simulink model "SF107A_MotRplCoggCmd"  (R2013b)
settings: Solver=FixedStepDiscrete  SolverMode=SingleTasking  StartTime=0.0  StopTime=1  FixedStep=0.002  RelTol=1e-3
values from neighbouring files (symbols this model uses):
  ARCHGLBPRM_2PI_ULS_F32 = DataDict.Constant    [SF107A_MotRplCoggCmd_DataDict.m]
  ARCHGLBPRM_FLOATZEROTHD_ULS_F32 = DataDict.Constant    [SF107A_MotRplCoggCmd_DataDict.m]
  ININITRNIDXCON_CNT_U16 = DataDict.Constant    [SF107A_MotRplCoggCmd_DataDict.m]
  ITRNIDXCON_CNT_U08 = DataDict.Constant    [SF107A_MotRplCoggCmd_DataDict.m]
  MotRplCoggCmdHrmncOrder1Elec = DataDict.Calibration    [SF107A_MotRplCoggCmd_DataDict.m]
  MotRplCoggCmdHrmncOrder2Elec = DataDict.Calibration    [SF107A_MotRplCoggCmd_DataDict.m]
  MotRplCoggCmdHrmncOrder3Elec = DataDict.Calibration    [SF107A_MotRplCoggCmd_DataDict.m]
  ONEOVER12_MOTREV_F32 = DataDict.Constant    [SF107A_MotRplCoggCmd_DataDict.m]
  ONEOVER2_ULS_F32 = DataDict.Constant    [SF107A_MotRplCoggCmd_DataDict.m]
  ONEOVER2PI_ULS_F32 = DataDict.Constant    [SF107A_MotRplCoggCmd_DataDict.m]
  ONEOVER4_ULS_F32 = DataDict.Constant    [SF107A_MotRplCoggCmd_DataDict.m]
  SINCNVNCON1_ULS_F32 = DataDict.Constant    [SF107A_MotRplCoggCmd_DataDict.m]
  SINCNVNCON2_ULS_F32 = DataDict.Constant    [SF107A_MotRplCoggCmd_DataDict.m]
  SINCNVNCONTBL_ULS_U16 = DataDict.Constant    [SF107A_MotRplCoggCmd_DataDict.m]
undefined symbols (not defined in the file or in its folder): NvmGetErrSts1
libraries: FloatToFixd x8, FixdToFloat x8, NxtrNvM x3, NxtrLim x3, simulink x2, NxtrAbslt x1
(part 2 of 3)

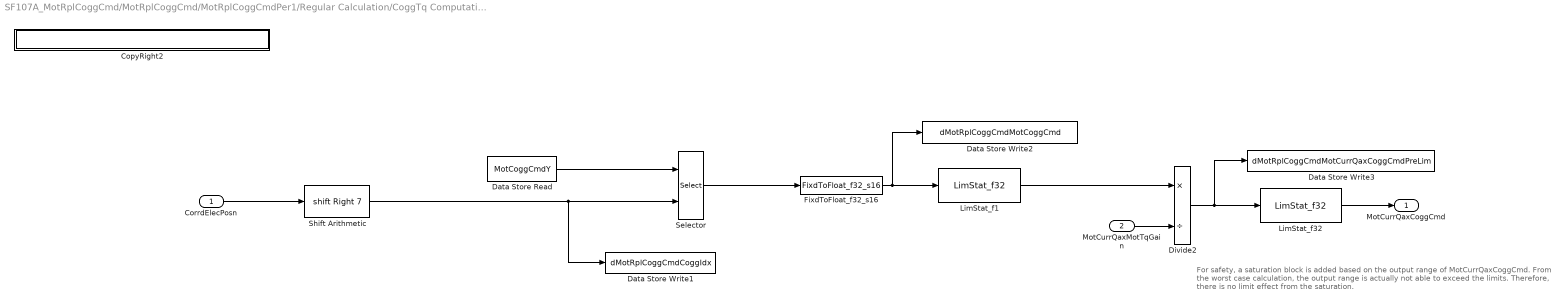
== system SF107A_MotRplCoggCmd/MotRplCoggCmd/MotRplCoggCmdPer1/Regular Calculation/CoggTq Computation ==
  note: For safety, a saturation block is added based on the output range of MotCurrQaxCoggCmd.
      | From the worst case calculation, the output range is actually not able to exceed the limits.
      | Therefore, there is no limit effect from the saturation.
  CorrdElecPosn : Inport
  MotCurrQaxMotTqGain : Inport  Port=2
  CopyRight2 : Subsystem  Description=|  mask(Copyright Information){none=on}
      | Copyright info block.                                               
      |                                                                     
      | Place copyright information at the top of every subsystem in design.
      mask prompts: none "No parameters"
      mask help: Place copyright information at the top of every subsystem in design.
      mask Display:
      | NxtrConf = 'Nexteer Confidential';
      | 
      | sys = bdroot; %handle for the current model ("system")
      | first = get_param(sys,'Created');
      | if(isempty(first))
      |     first = datestr(now,'yyyy');
      | else
      |     first = first(end-3:end);  %year is last four digits
      | end
      | 
      | last = get_param(sys,'LastModifiedDate');
      | if isempty(last)
      |     last = datestr(now,'yyyy');
      | else
      |     last = last(end-3:end);
      | end
      | 
      | if strcmp(first,last)
      |     fprintf('%s -- Copyright %s Nexteer',NxtrConf,first)
      | else
      |     fprintf('%s -- %s%s- %s Nexteer',NxtrConf,char(169),first,last)
      | end
  Data Store Read : DataStoreRead  RequirementInfo="{'linktype_rmi_doors' '0000bb46 (/E-STEER Core/SubSystem Specifications/Application Functions/SF99/SF107A Cogging and Ripple Command Generation)' '#SF107A_56' 'true' 'REQ:  SF107A_56' '' } %GIDa_3e95ac0e_f3f3_418f_9ebe_c4c5a1a291e1"  DataStoreName=MotCoggCmdY
  Data Store Write1 : DataStoreWrite  DataStoreName=dMotRplCoggCmdCoggIdx
  Data Store Write2 : DataStoreWrite  DataStoreName=dMotRplCoggCmdMotCoggCmd
  Data Store Write3 : DataStoreWrite  DataStoreName=dMotRplCoggCmdMotCurrQaxCoggCmdPreLim
  Divide2 : Product  RequirementInfo="{'linktype_rmi_doors' '0000bb46 (/E-STEER Core/SubSystem Specifications/Application Functions/SF99/SF107A Cogging and Ripple Command Generation)' '#SF107A_59' 'true' 'REQ:  SF107A_59' '' } %GIDa_3d8574ba_c11a_41bc_960f_b43c967fb16a"  Inputs=*/
  FixdToFloat_f32_s16 : FixdToFloat/FixdToFloat_f32_s16  Param1=14
  LimStat_f1 : NxtrLim/LimStat_f32  RequirementInfo="{'linktype_rmi_doors' '0000bb46 (/E-STEER Core/SubSystem Specifications/Application Functions/SF99/SF107A Cogging and Ripple Command Generation)' '#SF107A_52' 'true' 'REQ:  SF107A_52' '' } %GIDa_e794c357_2251_4144_9bb5_41f34ca7d615"  LoLim=MOTCOGGCMDLOLIM_MOTNWTMTR_F32  HiLim=MOTCOGGCMDHILIM_MOTNWTMTR_F32
      settings: AttributesFormatString=|
      | Low Limit: %<LoLim>
      | High Limit:%<HiLim>
  LimStat_f32 : NxtrLim/LimStat_f32  LoLim=MOTCURRCOGGCMDLOLIM_AMPR_F32  HiLim=MOTCURRCOGGCMDHILIM_AMPR_F32
      settings: AttributesFormatString=|
      | Low Limit: %<LoLim>
      | High Limit:%<HiLim>
  Selector : Selector  IndexMode=Zero-based  InputPortWidth=512  IndexOptions=Index vector (port)  Indices=[1 3]  OutputSizes=1
  Shift Arithmetic : ArithShift  BitShiftNumber=7  BitShiftDirection=Right
  MotCurrQaxCoggCmd : Outport
  wires:
  Selector/1 -> FixdToFloat_f32_s16/1
  FixdToFloat_f32_s16/1 -> LimStat_f1/1, Data Store Write2/1
  Data Store Read/1 -> Selector/1
  CorrdElecPosn/1 -> Shift Arithmetic/1
  MotCurrQaxMotTqGain/1 -> Divide2/2
  Divide2/1 -> LimStat_f32/1, Data Store Write3/1
  LimStat_f32/1 -> MotCurrQaxCoggCmd/1
  LimStat_f1/1 -> Divide2/1
  Shift Arithmetic/1 -> Data Store Write1/1, Selector/2

== system SF107A_MotRplCoggCmd/MotRplCoggCmd/MotRplCoggCmdPer1/Regular Calculation/CopyRight2 ==

== system SF107A_MotRplCoggCmd/MotRplCoggCmd/MotRplCoggCmdPer1/Regular Calculation/MotElecMeclPolarity Compensating ==
  MotElecMeclPolarity : Inport
  CopyRight2 : Subsystem  Description=|  mask(Copyright Information){none=on}
      | Copyright info block.                                               
      |                                                                     
      | Place copyright information at the top of every subsystem in design.
      mask prompts: none "No parameters"
      mask help: Place copyright information at the top of every subsystem in design.
      mask Display:
      | NxtrConf = 'Nexteer Confidential';
      | 
      | sys = bdroot; %handle for the current model ("system")
      | first = get_param(sys,'Created');
      | if(isempty(first))
      |     first = datestr(now,'yyyy');
      | else
      |     first = first(end-3:end);  %year is last four digits
      | end
      | 
      | last = get_param(sys,'LastModifiedDate');
      | if isempty(last)
      |     last = datestr(now,'yyyy');
      | else
      |     last = last(end-3:end);
      | end
      | 
      | if strcmp(first,last)
      |     fprintf('%s -- Copyright %s Nexteer',NxtrConf,first)
      | else
      |     fprintf('%s -- %s%s- %s Nexteer',NxtrConf,char(169),first,last)
      | end
  If1 : If  RequirementInfo="{'linktype_rmi_doors' '0000bb46 (/E-STEER Core/SubSystem Specifications/Application Functions/SF99/SF107A Cogging and Ripple Command Generation)' '#SF107A_48' 'true' 'REQ:  SF107A_48' '' } %GIDa_a3654d20_efbd_409e_83f9_fffa28f30d15"  IfExpression=u1==1
  Merge1 : Merge  RequirementInfo="{'linktype_rmi_doors' '0000bb46 (/E-STEER Core/SubSystem Specifications/Application Functions/SF99/SF107A Cogging and Ripple Command Generation)' '#SF107A_48' 'true' 'REQ:  SF107A_48' '' } %GIDa_23ad6171_7acd_41c2_a6a2_32a771c6a2a5"
  Output -1/12 MotRev : Subsystem  RequirementInfo="{'linktype_rmi_doors' '0000bb46 (/E-STEER Core/SubSystem Specifications/Application Functions/SF99/SF107A Cogging and Ripple Command Generation)' '#SF107A_48' 'true' 'REQ:  SF107A_48' '' } %GIDa_8d1ad6c2_c515_4934_932f_4d33d8ad8416"  TreatAsAtomicUnit=on
  Output 1/12 MotRev : Subsystem  RequirementInfo="{'linktype_rmi_doors' '0000bb46 (/E-STEER Core/SubSystem Specifications/Application Functions/SF99/SF107A Cogging and Ripple Command Generation)' '#SF107A_48' 'true' 'REQ:  SF107A_48' '' } %GIDa_3ad96f2a_4308_4c62_b762_7be6e9bb4790"  TreatAsAtomicUnit=on
  MotElecMeclPolarityCmp : Outport
  wires:
  If1/2 -> Output 1/12 MotRev/Action
  MotElecMeclPolarity/1 -> If1/1
  Merge1/1 -> MotElecMeclPolarityCmp/1
  Output -1/12 MotRev/1(Out1) -> Merge1/1
  If1/1 -> Output -1/12 MotRev/Action
  Output 1/12 MotRev/1(Out1) -> Merge1/2

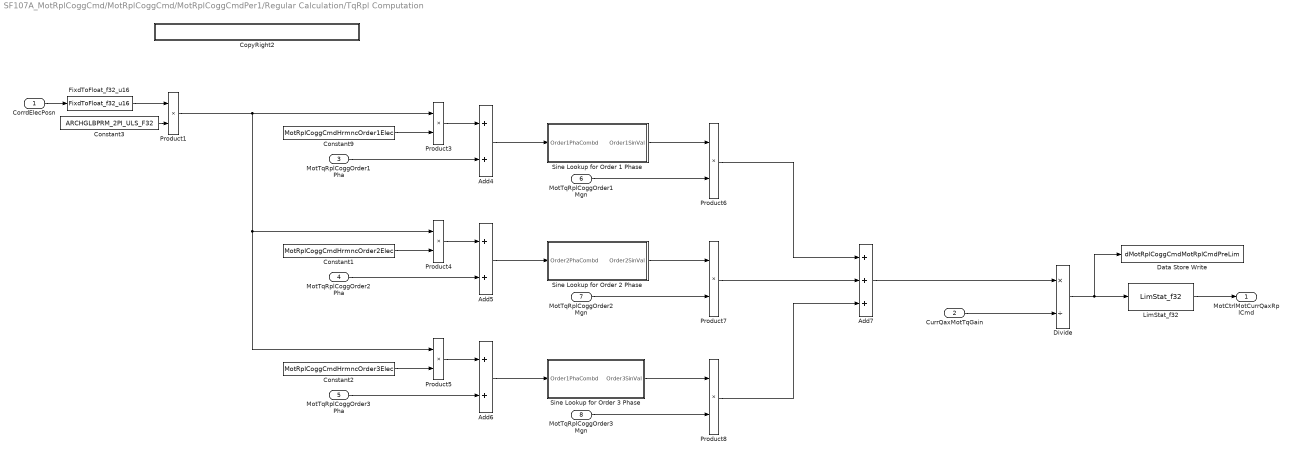
== system SF107A_MotRplCoggCmd/MotRplCoggCmd/MotRplCoggCmdPer1/Regular Calculation/TqRpl Computation ==
  CorrdElecPosn : Inport
  CurrQaxMotTqGain : Inport  Port=2
  MotTqRplCoggOrder1Pha : Inport  Port=3
  MotTqRplCoggOrder2Pha : Inport  Port=4
  MotTqRplCoggOrder3Pha : Inport  Port=5
  MotTqRplCoggOrder1Mgn : Inport  Port=6
  MotTqRplCoggOrder2Mgn : Inport  Port=7
  MotTqRplCoggOrder3Mgn : Inport  Port=8
  Add4 : Sum  RequirementInfo="{'linktype_rmi_doors' '0000bb46 (/E-STEER Core/SubSystem Specifications/Application Functions/SF99/SF107A Cogging and Ripple Command Generation)' '#SF107A_55' 'true' 'REQ:  SF107A_55' '' } %GIDa_c2399abb_93fd_4ea1_98cc_b0680e968892"
  Add5 : Sum  RequirementInfo="{'linktype_rmi_doors' '0000bb46 (/E-STEER Core/SubSystem Specifications/Application Functions/SF99/SF107A Cogging and Ripple Command Generation)' '#SF107A_55' 'true' 'REQ:  SF107A_55' '' } %GIDa_b4420672_1f55_4f94_87a8_96d9d357a965"
  Add6 : Sum  RequirementInfo="{'linktype_rmi_doors' '0000bb46 (/E-STEER Core/SubSystem Specifications/Application Functions/SF99/SF107A Cogging and Ripple Command Generation)' '#SF107A_55' 'true' 'REQ:  SF107A_55' '' } %GIDa_2dfbb206_2493_4fc1_9000_00a8fdd76cd7"
  Add7 : Sum  RequirementInfo="{'linktype_rmi_doors' '0000bb46 (/E-STEER Core/SubSystem Specifications/Application Functions/SF99/SF107A Cogging and Ripple Command Generation)' '#SF107A_54' 'true' 'REQ:  SF107A_54' '' } %GIDa_a8f048de_6f77_4343_a15f_fc7051edaaac"  Inputs=+++
  Constant1 : Constant  RequirementInfo="{'linktype_rmi_doors' '0000bb46 (/E-STEER Core/SubSystem Specifications/Application Functions/SF99/SF107A Cogging and Ripple Command Generation)' '#SF107A_57' 'true' 'REQ:  SF107A_57' '' } %GIDa_b7ef4c69_0a2c_4e9d_b8a7_dfaab4ba9f27"  Value=MotRplCoggCmdHrmncOrder2Elec
  Constant2 : Constant  RequirementInfo="{'linktype_rmi_doors' '0000bb46 (/E-STEER Core/SubSystem Specifications/Application Functions/SF99/SF107A Cogging and Ripple Command Generation)' '#SF107A_57' 'true' 'REQ:  SF107A_57' '' } %GIDa_07332141_8940_47cd_a6c0_7085309b4753"  Value=MotRplCoggCmdHrmncOrder3Elec
  Constant3 : Constant  Value=ARCHGLBPRM_2PI_ULS_F32
  Constant9 : Constant  RequirementInfo="{'linktype_rmi_doors' '0000bb46 (/E-STEER Core/SubSystem Specifications/Application Functions/SF99/SF107A Cogging and Ripple Command Generation)' '#SF107A_57' 'true' 'REQ:  SF107A_57' '' } %GIDa_3c0a14e8_7767_4d2c_90ce_8f5a73270d9c"  Value=MotRplCoggCmdHrmncOrder1Elec
  CopyRight2 : Subsystem  Description=|  mask(Copyright Information){none=on}
      | Copyright info block.                                               
      |                                                                     
      | Place copyright information at the top of every subsystem in design.
      mask prompts: none "No parameters"
      mask help: Place copyright information at the top of every subsystem in design.
      mask Display:
      | NxtrConf = 'Nexteer Confidential';
      | 
      | sys = bdroot; %handle for the current model ("system")
      | first = get_param(sys,'Created');
      | if(isempty(first))
      |     first = datestr(now,'yyyy');
      | else
      |     first = first(end-3:end);  %year is last four digits
      | end
      | 
      | last = get_param(sys,'LastModifiedDate');
      | if isempty(last)
      |     last = datestr(now,'yyyy');
      | else
      |     last = last(end-3:end);
      | end
      | 
      | if strcmp(first,last)
      |     fprintf('%s -- Copyright %s Nexteer',NxtrConf,first)
      | else
      |     fprintf('%s -- %s%s- %s Nexteer',NxtrConf,char(169),first,last)
      | end
  Data Store Write : DataStoreWrite  DataStoreName=dMotRplCoggCmdMotRplCmdPreLim
  Divide : Product  RequirementInfo="{'linktype_rmi_doors' '0000bb46 (/E-STEER Core/SubSystem Specifications/Application Functions/SF99/SF107A Cogging and Ripple Command Generation)' '#SF107A_53' 'true' 'REQ:  SF107A_53' '' } %GIDa_9f56ecef_e0c7_4e4a_ab4c_0d70a2d29558"  Inputs=*/
  FixdToFloat_f32_u16 : FixdToFloat/FixdToFloat_f32_u16  Param1=16
  LimStat_f32 : NxtrLim/LimStat_f32  LoLim=MOTRPLCMDLOLIM_AMPR_F32  HiLim=MOTRPLCMDHILIM_AMPR_F32
      settings: AttributesFormatString=|
      | Low Limit: %<LoLim>
      | High Limit:%<HiLim>
  Product1 : Product  RequirementInfo="{'linktype_rmi_doors' '0000bb46 (/E-STEER Core/SubSystem Specifications/Application Functions/SF99/SF107A Cogging and Ripple Command Generation)' '#SF107A_55' 'true' 'REQ:  SF107A_55' '' } %GIDa_8be27b70_a591_415b_b0b6_be9767e7231d"
  Product3 : Product  RequirementInfo="{'linktype_rmi_doors' '0000bb46 (/E-STEER Core/SubSystem Specifications/Application Functions/SF99/SF107A Cogging and Ripple Command Generation)' '#SF107A_55' 'true' 'REQ:  SF107A_55' '' } %GIDa_dd8066b3_0179_4f2f_b312_accdda934f40"
  Product4 : Product  RequirementInfo="{'linktype_rmi_doors' '0000bb46 (/E-STEER Core/SubSystem Specifications/Application Functions/SF99/SF107A Cogging and Ripple Command Generation)' '#SF107A_55' 'true' 'REQ:  SF107A_55' '' } %GIDa_811bec18_a835_44a9_8776_d6216b98e5e5"
  Product5 : Product  RequirementInfo="{'linktype_rmi_doors' '0000bb46 (/E-STEER Core/SubSystem Specifications/Application Functions/SF99/SF107A Cogging and Ripple Command Generation)' '#SF107A_55' 'true' 'REQ:  SF107A_55' '' } %GIDa_a9f9a7c0_debf_4fae_9cf4_183d284e7007"
  Product6 : Product  RequirementInfo="{'linktype_rmi_doors' '0000bb46 (/E-STEER Core/SubSystem Specifications/Application Functions/SF99/SF107A Cogging and Ripple Command Generation)' '#SF107A_55' 'true' 'REQ:  SF107A_55' '' } %GIDa_4a1c5c42_3c8b_4502_90cf_4cd7338fcd81"
  Product7 : Product  RequirementInfo="{'linktype_rmi_doors' '0000bb46 (/E-STEER Core/SubSystem Specifications/Application Functions/SF99/SF107A Cogging and Ripple Command Generation)' '#SF107A_55' 'true' 'REQ:  SF107A_55' '' } %GIDa_3d6707e5_ddb9_4eed_8831_c32e0231200b"
  Product8 : Product  RequirementInfo="{'linktype_rmi_doors' '0000bb46 (/E-STEER Core/SubSystem Specifications/Application Functions/SF99/SF107A Cogging and Ripple Command Generation)' '#SF107A_55' 'true' 'REQ:  SF107A_55' '' } %GIDa_09bf260f_b13c_4645_bce3_42c8e753e29d"
  Sine Lookup for Order 1 Phase : Subsystem  RequirementInfo="{'linktype_rmi_doors' '0000bb46 (/E-STEER Core/SubSystem Specifications/Application Functions/SF99/SF107A Cogging and Ripple Command Generation)' '#SF107A_55' 'true' 'REQ:  SF107A_55' '' } %GIDa_7a615d31_fc2b_4ba7_aa79_4cdec4c72968"
  Sine Lookup for Order 2 Phase : Subsystem  RequirementInfo="{'linktype_rmi_doors' '0000bb46 (/E-STEER Core/SubSystem Specifications/Application Functions/SF99/SF107A Cogging and Ripple Command Generation)' '#SF107A_55' 'true' 'REQ:  SF107A_55' '' } %GIDa_734c1328_0315_47be_ae6e_d11cd23f5817"
  Sine Lookup for Order 3 Phase : Subsystem  RequirementInfo="{'linktype_rmi_doors' '0000bb46 (/E-STEER Core/SubSystem Specifications/Application Functions/SF99/SF107A Cogging and Ripple Command Generation)' '#SF107A_55' 'true' 'REQ:  SF107A_55' '' } %GIDa_a57f7930_8d76_4290_b7d5_8e7d491e536a"
  MotCtrlMotCurrQaxRplCmd : Outport
  wires:
  Add6/1 -> Sine Lookup for Order 3 Phase/1(Order1PhaCombd)
  Product4/1 -> Add5/1
  Product6/1 -> Add7/1
  MotTqRplCoggOrder3Mgn/1 -> Product8/2
  Constant1/1 -> Product4/2
  Product3/1 -> Add4/1
  Add4/1 -> Sine Lookup for Order 1 Phase/1(Order1PhaCombd)
  MotTqRplCoggOrder2Mgn/1 -> Product7/2
  MotTqRplCoggOrder3Pha/1 -> Add6/2
  Sine Lookup for Order 2 Phase/1(Order2SinVal) -> Product7/1
  Add7/1 -> Divide/1
  Product8/1 -> Add7/3
  CorrdElecPosn/1 -> FixdToFloat_f32_u16/1
  Product5/1 -> Add6/1
  MotTqRplCoggOrder2Pha/1 -> Add5/2
  Constant2/1 -> Product5/2
  Sine Lookup for Order 1 Phase/1(Order1SinVal) -> Product6/1
  Product7/1 -> Add7/2
  Add5/1 -> Sine Lookup for Order 2 Phase/1(Order2PhaCombd)
  Divide/1 -> LimStat_f32/1, Data Store Write/1
  CurrQaxMotTqGain/1 -> Divide/2
  Constant9/1 -> Product3/2
  Sine Lookup for Order 3 Phase/1(Order3SinVal) -> Product8/1
  MotTqRplCoggOrder1Pha/1 -> Add4/2
  MotTqRplCoggOrder1Mgn/1 -> Product6/2
  LimStat_f32/1 -> MotCtrlMotCurrQaxRplCmd/1
  Product1/1 -> Product4/1, Product5/1, Product3/1
  FixdToFloat_f32_u16/1 -> Product1/1
  Constant3/1 -> Product1/2

== system SF107A_MotRplCoggCmd/MotRplCoggCmd/MotRplCoggCmdPer1/Set to 0/CopyRight2 ==

== system SF107A_MotRplCoggCmd/MotRplCoggCmd/SetMotCoggCmdPrm/For Iterator Subsystem1/CopyRight1 ==

== system SF107A_MotRplCoggCmd/MotRplCoggCmd/MotRplCoggCmdInit1/NVM is NOT okay/For Iterator Subsystem/CopyRight2 ==

== system SF107A_MotRplCoggCmd/MotRplCoggCmd/MotRplCoggCmdPer1/Regular Calculation/ Wrapping/CopyRight2 ==

== system SF107A_MotRplCoggCmd/MotRplCoggCmd/MotRplCoggCmdPer1/Regular Calculation/ Wrapping/If Action Subsystem1 ==
  Action Port : ActionPort  ActionType=then
  Constant : Constant  OutDataTypeStr=single
      settings: AttributesFormatString=%<OutDataTypeStr>
  CopyRight2 : Subsystem  Description=|  mask(Copyright Information){none=on}
      | Copyright info block.                                               
      |                                                                     
      | Place copyright information at the top of every subsystem in design.
      mask prompts: none "No parameters"
      mask help: Place copyright information at the top of every subsystem in design.
      mask Display:
      | NxtrConf = 'Nexteer Confidential';
      | 
      | sys = bdroot; %handle for the current model ("system")
      | first = get_param(sys,'Created');
      | if(isempty(first))
      |     first = datestr(now,'yyyy');
      | else
      |     first = first(end-3:end);  %year is last four digits
      | end
      | 
      | last = get_param(sys,'LastModifiedDate');
      | if isempty(last)
      |     last = datestr(now,'yyyy');
      | else
      |     last = last(end-3:end);
      | end
      | 
      | if strcmp(first,last)
      |     fprintf('%s -- Copyright %s Nexteer',NxtrConf,first)
      | else
      |     fprintf('%s -- %s%s- %s Nexteer',NxtrConf,char(169),first,last)
      | end
  Out1 : Outport
  wires:
  Constant/1 -> Out1/1

== system SF107A_MotRplCoggCmd/MotRplCoggCmd/MotRplCoggCmdPer1/Regular Calculation/ Wrapping/If Action Subsystem5 ==
  Action Port : ActionPort  ActionType=else
  Constant1 : Constant  Value=0  OutDataTypeStr=single
      settings: AttributesFormatString=%<OutDataTypeStr>
  CopyRight2 : Subsystem  Description=|  mask(Copyright Information){none=on}
      | Copyright info block.                                               
      |                                                                     
      | Place copyright information at the top of every subsystem in design.
      mask prompts: none "No parameters"
      mask help: Place copyright information at the top of every subsystem in design.
      mask Display:
      | NxtrConf = 'Nexteer Confidential';
      | 
      | sys = bdroot; %handle for the current model ("system")
      | first = get_param(sys,'Created');
      | if(isempty(first))
      |     first = datestr(now,'yyyy');
      | else
      |     first = first(end-3:end);  %year is last four digits
      | end
      | 
      | last = get_param(sys,'LastModifiedDate');
      | if isempty(last)
      |     last = datestr(now,'yyyy');
      | else
      |     last = last(end-3:end);
      | end
      | 
      | if strcmp(first,last)
      |     fprintf('%s -- Copyright %s Nexteer',NxtrConf,first)
      | else
      |     fprintf('%s -- %s%s- %s Nexteer',NxtrConf,char(169),first,last)
      | end
  Out1 : Outport
  wires:
  Constant1/1 -> Out1/1

== system SF107A_MotRplCoggCmd/MotRplCoggCmd/MotRplCoggCmdPer1/Regular Calculation/CoggTq Computation/CopyRight2 ==

== system SF107A_MotRplCoggCmd/MotRplCoggCmd/MotRplCoggCmdPer1/Regular Calculation/MotElecMeclPolarity Compensating/CopyRight2 ==

== system SF107A_MotRplCoggCmd/MotRplCoggCmd/MotRplCoggCmdPer1/Regular Calculation/MotElecMeclPolarity Compensating/Output -1//12 MotRev ==
  Action Port : ActionPort  ActionType=then
  Constant1 : Constant  Value=ONEOVER12_MOTREV_F32
  CopyRight2 : Subsystem  Description=|  mask(Copyright Information){none=on}
      | Copyright info block.                                               
      |                                                                     
      | Place copyright information at the top of every subsystem in design.
      mask prompts: none "No parameters"
      mask help: Place copyright information at the top of every subsystem in design.
      mask Display:
      | NxtrConf = 'Nexteer Confidential';
      | 
      | sys = bdroot; %handle for the current model ("system")
      | first = get_param(sys,'Created');
      | if(isempty(first))
      |     first = datestr(now,'yyyy');
      | else
      |     first = first(end-3:end);  %year is last four digits
      | end
      | 
      | last = get_param(sys,'LastModifiedDate');
      | if isempty(last)
      |     last = datestr(now,'yyyy');
      | else
      |     last = last(end-3:end);
      | end
      | 
      | if strcmp(first,last)
      |     fprintf('%s -- Copyright %s Nexteer',NxtrConf,first)
      | else
      |     fprintf('%s -- %s%s- %s Nexteer',NxtrConf,char(169),first,last)
      | end
  Unary Minus : UnaryMinus
  Out1 : Outport
  wires:
  Constant1/1 -> Unary Minus/1
  Unary Minus/1 -> Out1/1

== system SF107A_MotRplCoggCmd/MotRplCoggCmd/MotRplCoggCmdPer1/Regular Calculation/MotElecMeclPolarity Compensating/Output 1//12 MotRev ==
  Action Port : ActionPort  ActionType=else
  Constant1 : Constant  Value=ONEOVER12_MOTREV_F32
  CopyRight2 : Subsystem  Description=|  mask(Copyright Information){none=on}
      | Copyright info block.                                               
      |                                                                     
      | Place copyright information at the top of every subsystem in design.
      mask prompts: none "No parameters"
      mask help: Place copyright information at the top of every subsystem in design.
      mask Display:
      | NxtrConf = 'Nexteer Confidential';
      | 
      | sys = bdroot; %handle for the current model ("system")
      | first = get_param(sys,'Created');
      | if(isempty(first))
      |     first = datestr(now,'yyyy');
      | else
      |     first = first(end-3:end);  %year is last four digits
      | end
      | 
      | last = get_param(sys,'LastModifiedDate');
      | if isempty(last)
      |     last = datestr(now,'yyyy');
      | else
      |     last = last(end-3:end);
      | end
      | 
      | if strcmp(first,last)
      |     fprintf('%s -- Copyright %s Nexteer',NxtrConf,first)
      | else
      |     fprintf('%s -- %s%s- %s Nexteer',NxtrConf,char(169),first,last)
      | end
  Out1 : Outport
  wires:
  Constant1/1 -> Out1/1

== system SF107A_MotRplCoggCmd/MotRplCoggCmd/MotRplCoggCmdPer1/Regular Calculation/TqRpl Computation/CopyRight2 ==

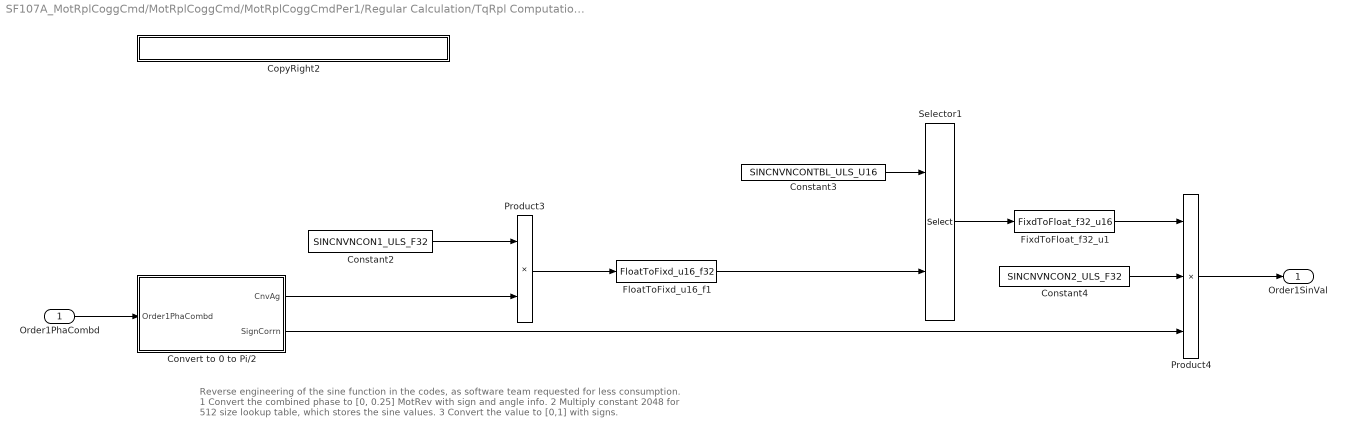
== system SF107A_MotRplCoggCmd/MotRplCoggCmd/MotRplCoggCmdPer1/Regular Calculation/TqRpl Computation/Sine Lookup for Order 1 Phase ==
  note: Reverse engineering of the sine function in the codes, as software team requested for less consumption.
      | 1 Convert the combined phase to [0, 0.25] MotRev with sign and angle info.
      | 2 Multiply constant 2048 for 512 size lookup table, which stores the sine values.
      | 3 Convert the value to [0,1] with signs.
  Order1PhaCombd : Inport
  Constant2 : Constant  Value=SINCNVNCON1_ULS_F32
  Constant3 : Constant  Value=SINCNVNCONTBL_ULS_U16
  Constant4 : Constant  Value=SINCNVNCON2_ULS_F32
  Convert to 0 to Pi/2 : Subsystem
  CopyRight2 : Subsystem  Description=|  mask(Copyright Information){none=on}
      | Copyright info block.                                               
      |                                                                     
      | Place copyright information at the top of every subsystem in design.
      mask prompts: none "No parameters"
      mask help: Place copyright information at the top of every subsystem in design.
      mask Display:
      | NxtrConf = 'Nexteer Confidential';
      | 
      | sys = bdroot; %handle for the current model ("system")
      | first = get_param(sys,'Created');
      | if(isempty(first))
      |     first = datestr(now,'yyyy');
      | else
      |     first = first(end-3:end);  %year is last four digits
      | end
      | 
      | last = get_param(sys,'LastModifiedDate');
      | if isempty(last)
      |     last = datestr(now,'yyyy');
      | else
      |     last = last(end-3:end);
      | end
      | 
      | if strcmp(first,last)
      |     fprintf('%s -- Copyright %s Nexteer',NxtrConf,first)
      | else
      |     fprintf('%s -- %s%s- %s Nexteer',NxtrConf,char(169),first,last)
      | end
  FixdToFloat_f32_u1 : FixdToFloat/FixdToFloat_f32_u16  Param1=0
  FloatToFixd_u16_f1 : FloatToFixd/FloatToFixd_u16_f32  Param1=0
  Product3 : Product
  Product4 : Product  Inputs=3
  Selector1 : Selector  IndexMode=Zero-based  InputPortWidth=513  IndexOptions=Index vector (port)  Indices=[1 3]  OutputSizes=1
  Order1SinVal : Outport
  wires:
  Product4/1 -> Order1SinVal/1
  FixdToFloat_f32_u1/1 -> Product4/1
  Constant4/1 -> Product4/2
  Selector1/1 -> FixdToFloat_f32_u1/1
  Product3/1 -> FloatToFixd_u16_f1/1
  Constant2/1 -> Product3/1
  Constant3/1 -> Selector1/1
  Order1PhaCombd/1 -> Convert to 0 to Pi/2/1(Order1PhaCombd)
  Convert to 0 to Pi/2/1(CnvAg) -> Product3/2
  Convert to 0 to Pi/2/2(SignCorrn) -> Product4/3
  FloatToFixd_u16_f1/1 -> Selector1/2

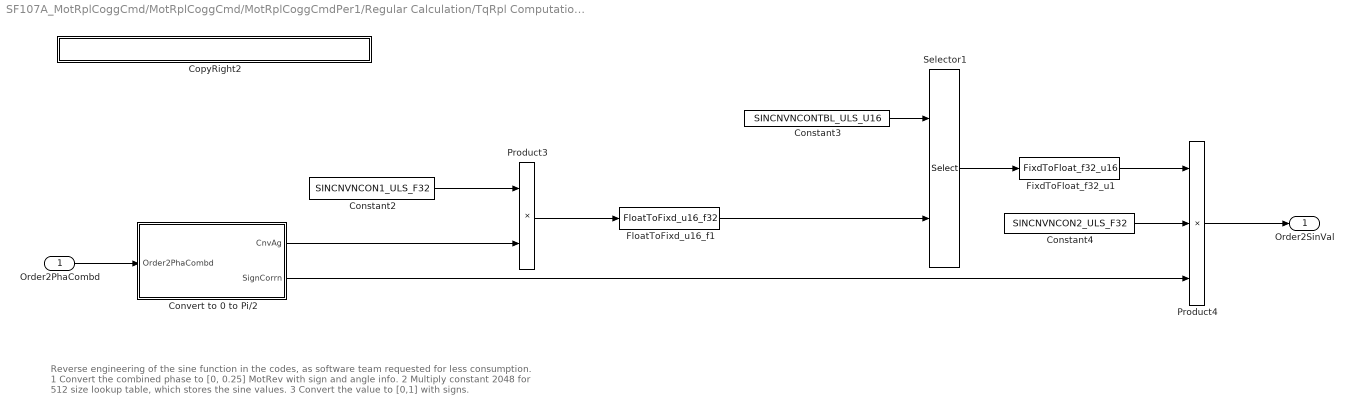
== system SF107A_MotRplCoggCmd/MotRplCoggCmd/MotRplCoggCmdPer1/Regular Calculation/TqRpl Computation/Sine Lookup for Order 2 Phase ==
  note: Reverse engineering of the sine function in the codes, as software team requested for less consumption.
      | 1 Convert the combined phase to [0, 0.25] MotRev with sign and angle info.
      | 2 Multiply constant 2048 for 512 size lookup table, which stores the sine values.
      | 3 Convert the value to [0,1] with signs.
  Order2PhaCombd : Inport
  Constant2 : Constant  Value=SINCNVNCON1_ULS_F32
  Constant3 : Constant  Value=SINCNVNCONTBL_ULS_U16
  Constant4 : Constant  Value=SINCNVNCON2_ULS_F32
  Convert to 0 to Pi/2 : Subsystem
  CopyRight2 : Subsystem  Description=|  mask(Copyright Information){none=on}
      | Copyright info block.                                               
      |                                                                     
      | Place copyright information at the top of every subsystem in design.
      mask prompts: none "No parameters"
      mask help: Place copyright information at the top of every subsystem in design.
      mask Display:
      | NxtrConf = 'Nexteer Confidential';
      | 
      | sys = bdroot; %handle for the current model ("system")
      | first = get_param(sys,'Created');
      | if(isempty(first))
      |     first = datestr(now,'yyyy');
      | else
      |     first = first(end-3:end);  %year is last four digits
      | end
      | 
      | last = get_param(sys,'LastModifiedDate');
      | if isempty(last)
      |     last = datestr(now,'yyyy');
      | else
      |     last = last(end-3:end);
      | end
      | 
      | if strcmp(first,last)
      |     fprintf('%s -- Copyright %s Nexteer',NxtrConf,first)
      | else
      |     fprintf('%s -- %s%s- %s Nexteer',NxtrConf,char(169),first,last)
      | end
  FixdToFloat_f32_u1 : FixdToFloat/FixdToFloat_f32_u16  Param1=0
  FloatToFixd_u16_f1 : FloatToFixd/FloatToFixd_u16_f32  Param1=0
  Product3 : Product
  Product4 : Product  Inputs=3
  Selector1 : Selector  IndexMode=Zero-based  InputPortWidth=513  IndexOptions=Index vector (port)  Indices=[1 3]  OutputSizes=1
  Order2SinVal : Outport
  wires:
  Convert to 0 to Pi/2/2(SignCorrn) -> Product4/3
  Convert to 0 to Pi/2/1(CnvAg) -> Product3/2
  Order2PhaCombd/1 -> Convert to 0 to Pi/2/1(Order2PhaCombd)
  Constant3/1 -> Selector1/1
  Constant2/1 -> Product3/1
  Product3/1 -> FloatToFixd_u16_f1/1
  FloatToFixd_u16_f1/1 -> Selector1/2
  Selector1/1 -> FixdToFloat_f32_u1/1
  Constant4/1 -> Product4/2
  FixdToFloat_f32_u1/1 -> Product4/1
  Product4/1 -> Order2SinVal/1

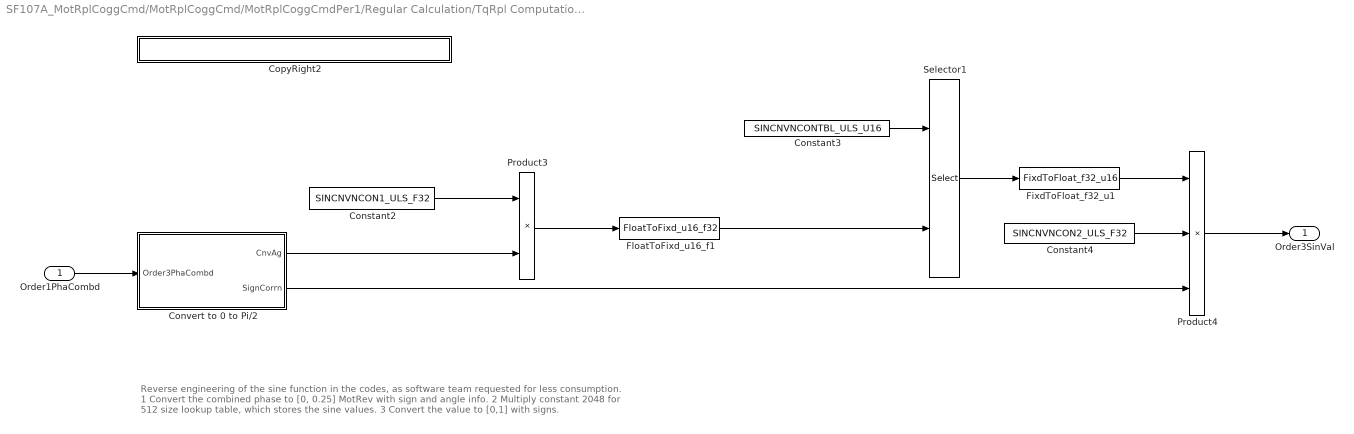
== system SF107A_MotRplCoggCmd/MotRplCoggCmd/MotRplCoggCmdPer1/Regular Calculation/TqRpl Computation/Sine Lookup for Order 3 Phase ==
  note: Reverse engineering of the sine function in the codes, as software team requested for less consumption.
      | 1 Convert the combined phase to [0, 0.25] MotRev with sign and angle info.
      | 2 Multiply constant 2048 for 512 size lookup table, which stores the sine values.
      | 3 Convert the value to [0,1] with signs.
  Order1PhaCombd : Inport
  Constant2 : Constant  Value=SINCNVNCON1_ULS_F32
  Constant3 : Constant  Value=SINCNVNCONTBL_ULS_U16
  Constant4 : Constant  Value=SINCNVNCON2_ULS_F32
  Convert to 0 to Pi/2 : Subsystem
  CopyRight2 : Subsystem  Description=|  mask(Copyright Information){none=on}
      | Copyright info block.                                               
      |                                                                     
      | Place copyright information at the top of every subsystem in design.
      mask prompts: none "No parameters"
      mask help: Place copyright information at the top of every subsystem in design.
      mask Display:
      | NxtrConf = 'Nexteer Confidential';
      | 
      | sys = bdroot; %handle for the current model ("system")
      | first = get_param(sys,'Created');
      | if(isempty(first))
      |     first = datestr(now,'yyyy');
      | else
      |     first = first(end-3:end);  %year is last four digits
      | end
      | 
      | last = get_param(sys,'LastModifiedDate');
      | if isempty(last)
      |     last = datestr(now,'yyyy');
      | else
      |     last = last(end-3:end);
      | end
      | 
      | if strcmp(first,last)
      |     fprintf('%s -- Copyright %s Nexteer',NxtrConf,first)
      | else
      |     fprintf('%s -- %s%s- %s Nexteer',NxtrConf,char(169),first,last)
      | end
  FixdToFloat_f32_u1 : FixdToFloat/FixdToFloat_f32_u16  Param1=0
  FloatToFixd_u16_f1 : FloatToFixd/FloatToFixd_u16_f32  Param1=0
  Product3 : Product
  Product4 : Product  Inputs=3
  Selector1 : Selector  IndexMode=Zero-based  InputPortWidth=513  IndexOptions=Index vector (port)  Indices=[1 3]  OutputSizes=1
  Order3SinVal : Outport
  wires:
  Product4/1 -> Order3SinVal/1
  FixdToFloat_f32_u1/1 -> Product4/1
  Constant4/1 -> Product4/2
  Selector1/1 -> FixdToFloat_f32_u1/1
  FloatToFixd_u16_f1/1 -> Selector1/2
  Product3/1 -> FloatToFixd_u16_f1/1
  Constant2/1 -> Product3/1
  Constant3/1 -> Selector1/1
  Order1PhaCombd/1 -> Convert to 0 to Pi/2/1(Order3PhaCombd)
  Convert to 0 to Pi/2/1(CnvAg) -> Product3/2
  Convert to 0 to Pi/2/2(SignCorrn) -> Product4/3

== system SF107A_MotRplCoggCmd/MotRplCoggCmd/MotRplCoggCmdPer1/Regular Calculation/ Wrapping/If Action Subsystem1/CopyRight2 ==

== system SF107A_MotRplCoggCmd/MotRplCoggCmd/MotRplCoggCmdPer1/Regular Calculation/ Wrapping/If Action Subsystem5/CopyRight2 ==

== system SF107A_MotRplCoggCmd/MotRplCoggCmd/MotRplCoggCmdPer1/Regular Calculation/MotElecMeclPolarity Compensating/Output -1//12 MotRev/CopyRight2 ==

== system SF107A_MotRplCoggCmd/MotRplCoggCmd/MotRplCoggCmdPer1/Regular Calculation/MotElecMeclPolarity Compensating/Output 1//12 MotRev/CopyRight2 ==

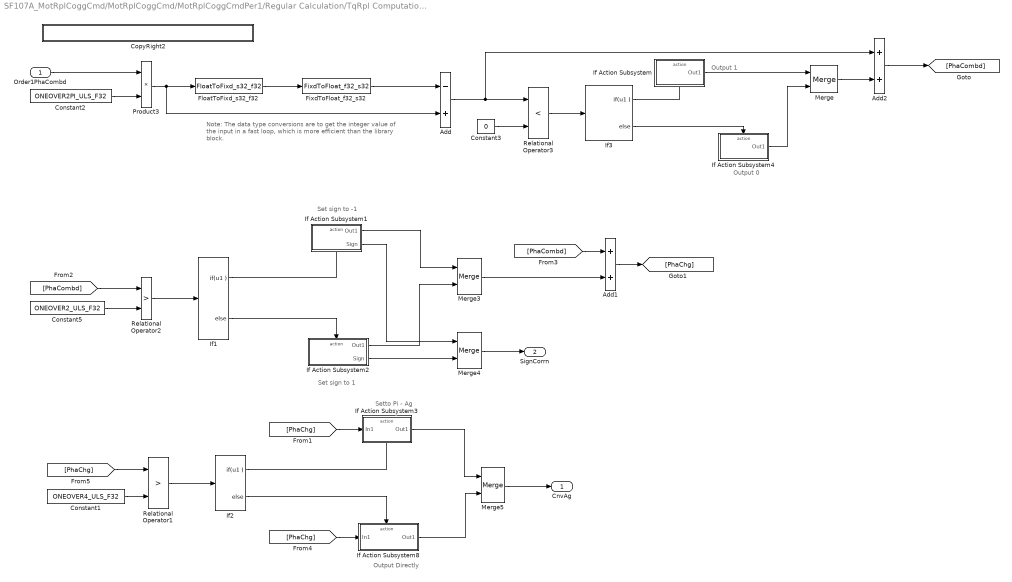
== system SF107A_MotRplCoggCmd/MotRplCoggCmd/MotRplCoggCmdPer1/Regular Calculation/TqRpl Computation/Sine Lookup for Order 1 Phase/Convert to 0 to Pi//2 ==
  note: Note: The data type conversions are to get the integer value of
      | the input in a fast loop, which is more efficient than the library
      | block.
  note: Output 1
  note: Output 0
  note: Output Directly
  note: Setto Pi - Ag
  note: Set sign to 1
  note: Set sign to -1
  Order1PhaCombd : Inport
  Add : Sum  Inputs=-+
  Add1 : Sum
  Add2 : Sum
  Constant1 : Constant  Value=ONEOVER4_ULS_F32
  Constant2 : Constant  Value=ONEOVER2PI_ULS_F32
  Constant3 : Constant  Value=0  OutDataTypeStr=single
      settings: AttributesFormatString=%<OutDataTypeStr>
  Constant5 : Constant  Value=ONEOVER2_ULS_F32
  CopyRight2 : Subsystem  Description=|  mask(Copyright Information){none=on}
      | Copyright info block.                                               
      |                                                                     
      | Place copyright information at the top of every subsystem in design.
      mask prompts: none "No parameters"
      mask help: Place copyright information at the top of every subsystem in design.
      mask Display:
      | NxtrConf = 'Nexteer Confidential';
      | 
      | sys = bdroot; %handle for the current model ("system")
      | first = get_param(sys,'Created');
      | if(isempty(first))
      |     first = datestr(now,'yyyy');
      | else
      |     first = first(end-3:end);  %year is last four digits
      | end
      | 
      | last = get_param(sys,'LastModifiedDate');
      | if isempty(last)
      |     last = datestr(now,'yyyy');
      | else
      |     last = last(end-3:end);
      | end
      | 
      | if strcmp(first,last)
      |     fprintf('%s -- Copyright %s Nexteer',NxtrConf,first)
      | else
      |     fprintf('%s -- %s%s- %s Nexteer',NxtrConf,char(169),first,last)
      | end
  FixdToFloat_f32_s32 : FixdToFloat/FixdToFloat_f32_s32  Param1=0
  FloatToFixd_s32_f32 : FloatToFixd/FloatToFixd_s32_f32  Param1=0
  If Action Subsystem : Subsystem  TreatAsAtomicUnit=on
  If Action Subsystem1 : Subsystem  TreatAsAtomicUnit=on
  If Action Subsystem2 : Subsystem  TreatAsAtomicUnit=on
  If Action Subsystem3 : Subsystem  TreatAsAtomicUnit=on
  If Action Subsystem4 : Subsystem  TreatAsAtomicUnit=on
  If Action Subsystem8 : Subsystem  TreatAsAtomicUnit=on
  If1 : If  IfExpression=u1
  If2 : If  IfExpression=u1
  If3 : If  IfExpression=u1
  Merge{,3..5} (4 alike) : Merge
  Product3 : Product
  Relational Operator1 : RelationalOperator  Operator=>  OutDataTypeStr=boolean
  Relational Operator2 : RelationalOperator  Operator=>  OutDataTypeStr=boolean
  Relational Operator3 : RelationalOperator  Operator=<  OutDataTypeStr=boolean
  CnvAg : Outport
  SignCorrn : Outport  Port=2
  wires:
  Merge4/1 -> SignCorrn/1
  Merge5/1 -> CnvAg/1
  If Action Subsystem2/2(Sign) -> Merge4/2
  Relational Operator1/1 -> If2/1
  [PhaCombd] -> Relational Operator2/1
  If2/1 -> If Action Subsystem3/Action
  Constant5/1 -> Relational Operator2/2
  [PhaCombd] -> Add1/1
  Merge3/1 -> Add1/2
  If2/2 -> If Action Subsystem8/Action
  If Action Subsystem1/1(Out1) -> Merge3/1
  If Action Subsystem2/1(Out1) -> Merge3/2
  [PhaChg] -> If Action Subsystem3/1(In1)
  If1/1 -> If Action Subsystem1/Action
  If Action Subsystem8/1(Out1) -> Merge5/2
  Add1/1 -> [PhaChg]
  If Action Subsystem1/2(Sign) -> Merge4/1
  If Action Subsystem3/1(Out1) -> Merge5/1
  Constant1/1 -> Relational Operator1/2
  If1/2 -> If Action Subsystem2/Action
  Relational Operator2/1 -> If1/1
  Order1PhaCombd/1 -> Product3/1
  Product3/1 -> Add/2, FloatToFixd_s32_f32/1
  Constant2/1 -> Product3/2
  [PhaChg] -> If Action Subsystem8/1(In1)
  [PhaChg] -> Relational Operator1/1
  FloatToFixd_s32_f32/1 -> FixdToFloat_f32_s32/1
  FixdToFloat_f32_s32/1 -> Add/1
  Add/1 -> Add2/1, Relational Operator3/1
  Relational Operator3/1 -> If3/1
  Constant3/1 -> Relational Operator3/2
  If3/1 -> If Action Subsystem/Action
  If3/2 -> If Action Subsystem4/Action
  If Action Subsystem/1(Out1) -> Merge/1
  If Action Subsystem4/1(Out1) -> Merge/2
  Add2/1 -> [PhaCombd]
  Merge/1 -> Add2/2

== system SF107A_MotRplCoggCmd/MotRplCoggCmd/MotRplCoggCmdPer1/Regular Calculation/TqRpl Computation/Sine Lookup for Order 1 Phase/CopyRight2 ==

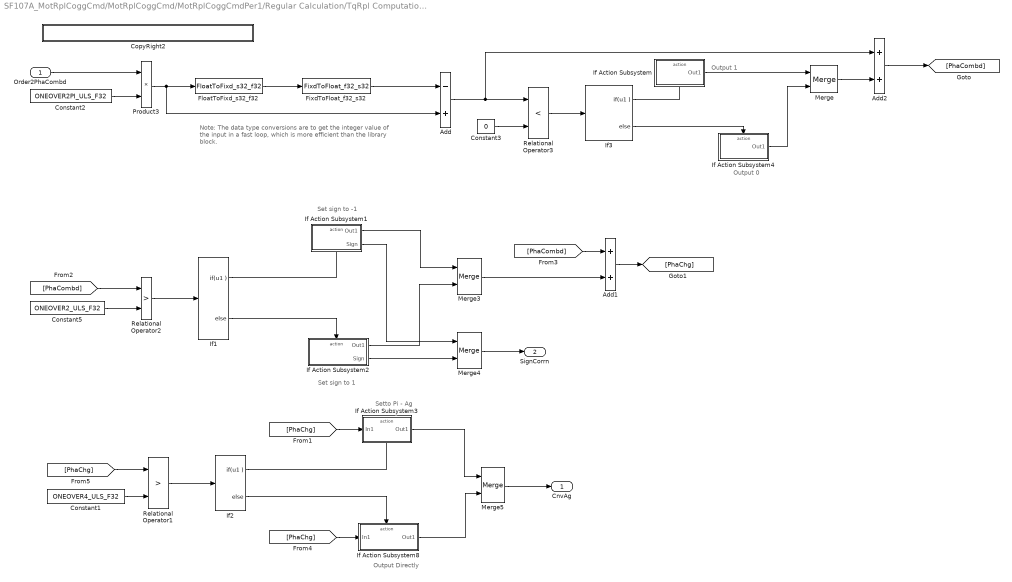
== system SF107A_MotRplCoggCmd/MotRplCoggCmd/MotRplCoggCmdPer1/Regular Calculation/TqRpl Computation/Sine Lookup for Order 2 Phase/Convert to 0 to Pi//2 ==
  note: Output 1
  note: Output 0
  note: Output Directly
  note: Setto Pi - Ag
  note: Set sign to 1
  note: Set sign to -1
  note: Note: The data type conversions are to get the integer value of
      | the input in a fast loop, which is more efficient than the library
      | block.
  Order2PhaCombd : Inport
  Add : Sum  Inputs=-+
  Add1 : Sum
  Add2 : Sum
  Constant1 : Constant  Value=ONEOVER4_ULS_F32
  Constant2 : Constant  Value=ONEOVER2PI_ULS_F32
  Constant3 : Constant  Value=0  OutDataTypeStr=single
      settings: AttributesFormatString=%<OutDataTypeStr>
  Constant5 : Constant  Value=ONEOVER2_ULS_F32
  CopyRight2 : Subsystem  Description=|  mask(Copyright Information){none=on}
      | Copyright info block.                                               
      |                                                                     
      | Place copyright information at the top of every subsystem in design.
      mask prompts: none "No parameters"
      mask help: Place copyright information at the top of every subsystem in design.
      mask Display:
      | NxtrConf = 'Nexteer Confidential';
      | 
      | sys = bdroot; %handle for the current model ("system")
      | first = get_param(sys,'Created');
      | if(isempty(first))
      |     first = datestr(now,'yyyy');
      | else
      |     first = first(end-3:end);  %year is last four digits
      | end
      | 
      | last = get_param(sys,'LastModifiedDate');
      | if isempty(last)
      |     last = datestr(now,'yyyy');
      | else
      |     last = last(end-3:end);
      | end
      | 
      | if strcmp(first,last)
      |     fprintf('%s -- Copyright %s Nexteer',NxtrConf,first)
      | else
      |     fprintf('%s -- %s%s- %s Nexteer',NxtrConf,char(169),first,last)
      | end
  FixdToFloat_f32_s32 : FixdToFloat/FixdToFloat_f32_s32  Param1=0
  FloatToFixd_s32_f32 : FloatToFixd/FloatToFixd_s32_f32  Param1=0
  If Action Subsystem : Subsystem  TreatAsAtomicUnit=on
  If Action Subsystem1 : Subsystem  TreatAsAtomicUnit=on
  If Action Subsystem2 : Subsystem  TreatAsAtomicUnit=on
  If Action Subsystem3 : Subsystem  TreatAsAtomicUnit=on
  If Action Subsystem4 : Subsystem  TreatAsAtomicUnit=on
  If Action Subsystem8 : Subsystem  TreatAsAtomicUnit=on
  If1 : If  IfExpression=u1
  If2 : If  IfExpression=u1
  If3 : If  IfExpression=u1
  Merge{,3..5} (4 alike) : Merge
  Product3 : Product
  Relational Operator1 : RelationalOperator  Operator=>  OutDataTypeStr=boolean
  Relational Operator2 : RelationalOperator  Operator=>  OutDataTypeStr=boolean
  Relational Operator3 : RelationalOperator  Operator=<  OutDataTypeStr=boolean
  CnvAg : Outport
  SignCorrn : Outport  Port=2
  wires:
  Merge4/1 -> SignCorrn/1
  Merge5/1 -> CnvAg/1
  If Action Subsystem2/2(Sign) -> Merge4/2
  Relational Operator1/1 -> If2/1
  [PhaCombd] -> Relational Operator2/1
  If2/1 -> If Action Subsystem3/Action
  Constant5/1 -> Relational Operator2/2
  [PhaCombd] -> Add1/1
  Merge3/1 -> Add1/2
  If2/2 -> If Action Subsystem8/Action
  If Action Subsystem1/1(Out1) -> Merge3/1
  If Action Subsystem2/1(Out1) -> Merge3/2
  [PhaChg] -> If Action Subsystem3/1(In1)
  If1/1 -> If Action Subsystem1/Action
  If Action Subsystem8/1(Out1) -> Merge5/2
  Add1/1 -> [PhaChg]
  If Action Subsystem1/2(Sign) -> Merge4/1
  If Action Subsystem3/1(Out1) -> Merge5/1
  Constant1/1 -> Relational Operator1/2
  If1/2 -> If Action Subsystem2/Action
  Relational Operator2/1 -> If1/1
  Order2PhaCombd/1 -> Product3/1
  Product3/1 -> Add/2, FloatToFixd_s32_f32/1
  Constant2/1 -> Product3/2
  [PhaChg] -> If Action Subsystem8/1(In1)
  [PhaChg] -> Relational Operator1/1
  FloatToFixd_s32_f32/1 -> FixdToFloat_f32_s32/1
  FixdToFloat_f32_s32/1 -> Add/1
  Add/1 -> Add2/1, Relational Operator3/1
  Relational Operator3/1 -> If3/1
  Constant3/1 -> Relational Operator3/2
  If3/1 -> If Action Subsystem/Action
  If3/2 -> If Action Subsystem4/Action
  If Action Subsystem/1(Out1) -> Merge/1
  If Action Subsystem4/1(Out1) -> Merge/2
  Add2/1 -> [PhaCombd]
  Merge/1 -> Add2/2

== system SF107A_MotRplCoggCmd/MotRplCoggCmd/MotRplCoggCmdPer1/Regular Calculation/TqRpl Computation/Sine Lookup for Order 2 Phase/CopyRight2 ==

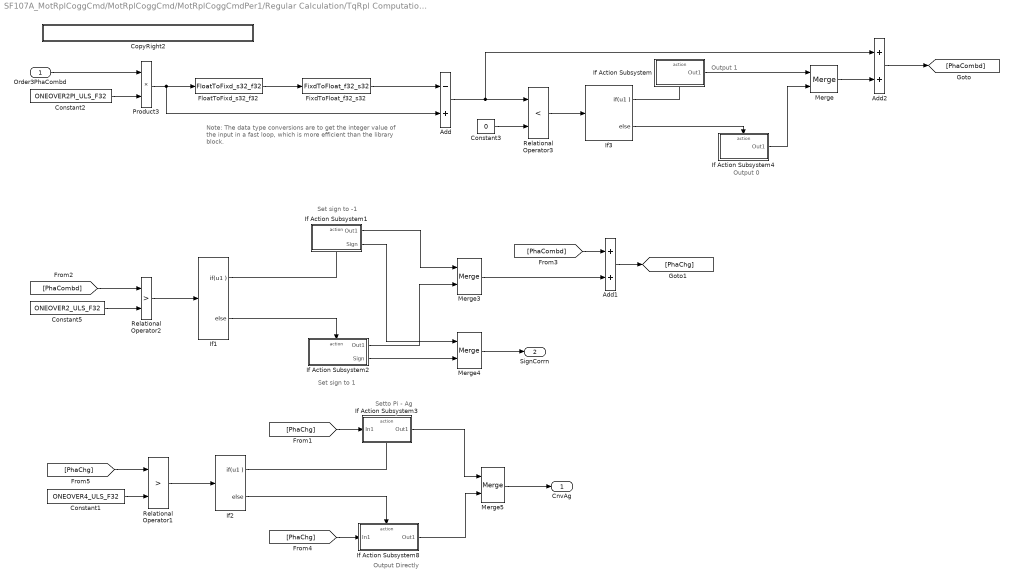
== system SF107A_MotRplCoggCmd/MotRplCoggCmd/MotRplCoggCmdPer1/Regular Calculation/TqRpl Computation/Sine Lookup for Order 3 Phase/Convert to 0 to Pi//2 ==
  note: Output 1
  note: Output 0
  note: Output Directly
  note: Setto Pi - Ag
  note: Set sign to 1
  note: Set sign to -1
  note: Note: The data type conversions are to get the integer value of
      | the input in a fast loop, which is more efficient than the library
      | block.
  Order3PhaCombd : Inport
  Add : Sum  Inputs=-+
  Add1 : Sum
  Add2 : Sum
  Constant1 : Constant  Value=ONEOVER4_ULS_F32
  Constant2 : Constant  Value=ONEOVER2PI_ULS_F32
  Constant3 : Constant  Value=0  OutDataTypeStr=single
      settings: AttributesFormatString=%<OutDataTypeStr>
  Constant5 : Constant  Value=ONEOVER2_ULS_F32
  CopyRight2 : Subsystem  Description=|  mask(Copyright Information){none=on}
      | Copyright info block.                                               
      |                                                                     
      | Place copyright information at the top of every subsystem in design.
      mask prompts: none "No parameters"
      mask help: Place copyright information at the top of every subsystem in design.
      mask Display:
      | NxtrConf = 'Nexteer Confidential';
      | 
      | sys = bdroot; %handle for the current model ("system")
      | first = get_param(sys,'Created');
      | if(isempty(first))
      |     first = datestr(now,'yyyy');
      | else
      |     first = first(end-3:end);  %year is last four digits
      | end
      | 
      | last = get_param(sys,'LastModifiedDate');
      | if isempty(last)
      |     last = datestr(now,'yyyy');
      | else
      |     last = last(end-3:end);
      | end
      | 
      | if strcmp(first,last)
      |     fprintf('%s -- Copyright %s Nexteer',NxtrConf,first)
      | else
      |     fprintf('%s -- %s%s- %s Nexteer',NxtrConf,char(169),first,last)
      | end
  FixdToFloat_f32_s32 : FixdToFloat/FixdToFloat_f32_s32  Param1=0
  FloatToFixd_s32_f32 : FloatToFixd/FloatToFixd_s32_f32  Param1=0
  If Action Subsystem : Subsystem  TreatAsAtomicUnit=on
  If Action Subsystem1 : Subsystem  TreatAsAtomicUnit=on
  If Action Subsystem2 : Subsystem  TreatAsAtomicUnit=on
  If Action Subsystem3 : Subsystem  TreatAsAtomicUnit=on
  If Action Subsystem4 : Subsystem  TreatAsAtomicUnit=on
  If Action Subsystem8 : Subsystem  TreatAsAtomicUnit=on
  If1 : If  IfExpression=u1
  If2 : If  IfExpression=u1
  If3 : If  IfExpression=u1
  Merge{,3..5} (4 alike) : Merge
  Product3 : Product
  Relational Operator1 : RelationalOperator  Operator=>  OutDataTypeStr=boolean
  Relational Operator2 : RelationalOperator  Operator=>  OutDataTypeStr=boolean
  Relational Operator3 : RelationalOperator  Operator=<  OutDataTypeStr=boolean
  CnvAg : Outport
  SignCorrn : Outport  Port=2
  wires:
  Merge4/1 -> SignCorrn/1
  Merge5/1 -> CnvAg/1
  If Action Subsystem2/2(Sign) -> Merge4/2
  Relational Operator1/1 -> If2/1
  [PhaCombd] -> Relational Operator2/1
  If2/1 -> If Action Subsystem3/Action
  Constant5/1 -> Relational Operator2/2
  [PhaCombd] -> Add1/1
  Merge3/1 -> Add1/2
  If2/2 -> If Action Subsystem8/Action
  If Action Subsystem1/1(Out1) -> Merge3/1
  If Action Subsystem2/1(Out1) -> Merge3/2
  [PhaChg] -> If Action Subsystem3/1(In1)
  If1/1 -> If Action Subsystem1/Action
  If Action Subsystem8/1(Out1) -> Merge5/2
  Add1/1 -> [PhaChg]
  If Action Subsystem1/2(Sign) -> Merge4/1
  If Action Subsystem3/1(Out1) -> Merge5/1
  Constant1/1 -> Relational Operator1/2
  If1/2 -> If Action Subsystem2/Action
  Relational Operator2/1 -> If1/1
  Order3PhaCombd/1 -> Product3/1
  Product3/1 -> Add/2, FloatToFixd_s32_f32/1
  Constant2/1 -> Product3/2
  [PhaChg] -> If Action Subsystem8/1(In1)
  [PhaChg] -> Relational Operator1/1
  FloatToFixd_s32_f32/1 -> FixdToFloat_f32_s32/1
  FixdToFloat_f32_s32/1 -> Add/1
  Add/1 -> Add2/1, Relational Operator3/1
  Relational Operator3/1 -> If3/1
  Constant3/1 -> Relational Operator3/2
  If3/1 -> If Action Subsystem/Action
  If3/2 -> If Action Subsystem4/Action
  If Action Subsystem/1(Out1) -> Merge/1
  If Action Subsystem4/1(Out1) -> Merge/2
  Add2/1 -> [PhaCombd]
  Merge/1 -> Add2/2

== system SF107A_MotRplCoggCmd/MotRplCoggCmd/MotRplCoggCmdPer1/Regular Calculation/TqRpl Computation/Sine Lookup for Order 3 Phase/CopyRight2 ==

== system SF107A_MotRplCoggCmd/MotRplCoggCmd/MotRplCoggCmdPer1/Regular Calculation/TqRpl Computation/Sine Lookup for Order 1 Phase/Convert to 0 to Pi//2/CopyRight2 ==

== system SF107A_MotRplCoggCmd/MotRplCoggCmd/MotRplCoggCmdPer1/Regular Calculation/TqRpl Computation/Sine Lookup for Order 1 Phase/Convert to 0 to Pi//2/If Action Subsystem ==
  Action Port : ActionPort  ActionType=then
  Constant3 : Constant  OutDataTypeStr=single
      settings: AttributesFormatString=%<OutDataTypeStr>
  CopyRight2 : Subsystem  Description=|  mask(Copyright Information){none=on}
      | Copyright info block.                                               
      |                                                                     
      | Place copyright information at the top of every subsystem in design.
      mask prompts: none "No parameters"
      mask help: Place copyright information at the top of every subsystem in design.
      mask Display:
      | NxtrConf = 'Nexteer Confidential';
      | 
      | sys = bdroot; %handle for the current model ("system")
      | first = get_param(sys,'Created');
      | if(isempty(first))
      |     first = datestr(now,'yyyy');
      | else
      |     first = first(end-3:end);  %year is last four digits
      | end
      | 
      | last = get_param(sys,'LastModifiedDate');
      | if isempty(last)
      |     last = datestr(now,'yyyy');
      | else
      |     last = last(end-3:end);
      | end
      | 
      | if strcmp(first,last)
      |     fprintf('%s -- Copyright %s Nexteer',NxtrConf,first)
      | else
      |     fprintf('%s -- %s%s- %s Nexteer',NxtrConf,char(169),first,last)
      | end
  Out1 : Outport
  wires:
  Constant3/1 -> Out1/1

== system SF107A_MotRplCoggCmd/MotRplCoggCmd/MotRplCoggCmdPer1/Regular Calculation/TqRpl Computation/Sine Lookup for Order 1 Phase/Convert to 0 to Pi//2/If Action Subsystem1 ==
  Action Port : ActionPort  ActionType=then
  Constant1 : Constant  OutDataTypeStr=single
      settings: AttributesFormatString=%<OutDataTypeStr>
  Constant2 : Constant  Value=ONEOVER2_ULS_F32
  CopyRight2 : Subsystem  Description=|  mask(Copyright Information){none=on}
      | Copyright info block.                                               
      |                                                                     
      | Place copyright information at the top of every subsystem in design.
      mask prompts: none "No parameters"
      mask help: Place copyright information at the top of every subsystem in design.
      mask Display:
      | NxtrConf = 'Nexteer Confidential';
      | 
      | sys = bdroot; %handle for the current model ("system")
      | first = get_param(sys,'Created');
      | if(isempty(first))
      |     first = datestr(now,'yyyy');
      | else
      |     first = first(end-3:end);  %year is last four digits
      | end
      | 
      | last = get_param(sys,'LastModifiedDate');
      | if isempty(last)
      |     last = datestr(now,'yyyy');
      | else
      |     last = last(end-3:end);
      | end
      | 
      | if strcmp(first,last)
      |     fprintf('%s -- Copyright %s Nexteer',NxtrConf,first)
      | else
      |     fprintf('%s -- %s%s- %s Nexteer',NxtrConf,char(169),first,last)
      | end
  Unary Minus : UnaryMinus
  Unary Minus1 : UnaryMinus
  Out1 : Outport
  Sign : Outport  Port=2
  wires:
  Constant1/1 -> Unary Minus1/1
  Constant2/1 -> Unary Minus/1
  Unary Minus/1 -> Out1/1
  Unary Minus1/1 -> Sign/1

== system SF107A_MotRplCoggCmd/MotRplCoggCmd/MotRplCoggCmdPer1/Regular Calculation/TqRpl Computation/Sine Lookup for Order 1 Phase/Convert to 0 to Pi//2/If Action Subsystem2 ==
  Action Port : ActionPort  ActionType=else
  Constant1 : Constant  OutDataTypeStr=single
      settings: AttributesFormatString=%<OutDataTypeStr>
  Constant2 : Constant  Value=0  OutDataTypeStr=single
      settings: AttributesFormatString=%<OutDataTypeStr>
  CopyRight2 : Subsystem  Description=|  mask(Copyright Information){none=on}
      | Copyright info block.                                               
      |                                                                     
      | Place copyright information at the top of every subsystem in design.
      mask prompts: none "No parameters"
      mask help: Place copyright information at the top of every subsystem in design.
      mask Display:
      | NxtrConf = 'Nexteer Confidential';
      | 
      | sys = bdroot; %handle for the current model ("system")
      | first = get_param(sys,'Created');
      | if(isempty(first))
      |     first = datestr(now,'yyyy');
      | else
      |     first = first(end-3:end);  %year is last four digits
      | end
      | 
      | last = get_param(sys,'LastModifiedDate');
      | if isempty(last)
      |     last = datestr(now,'yyyy');
      | else
      |     last = last(end-3:end);
      | end
      | 
      | if strcmp(first,last)
      |     fprintf('%s -- Copyright %s Nexteer',NxtrConf,first)
      | else
      |     fprintf('%s -- %s%s- %s Nexteer',NxtrConf,char(169),first,last)
      | end
  Out1 : Outport
  Sign : Outport  Port=2
  wires:
  Constant2/1 -> Out1/1
  Constant1/1 -> Sign/1
